simulink model "untitled"  (R2016b)
settings: Solver=VariableStepAuto  StartTime=0.0  StopTime=10.0  RelTol=1e-3
settings Model: Creator=drazz  LastModifiedBy=drazz

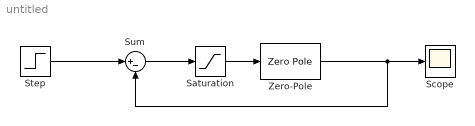
== system untitled ==
  Saturation : Saturate
  Scope : Scope
  Step : Step  SampleTime=0
  Sum : Sum  Inputs=|+-
  Zero-Pole : ZeroPole  Poles=[0 -1]
  wires:
  Zero-Pole/1 -> Sum/2, Scope/1
  Saturation/1 -> Zero-Pole/1
  Sum/1 -> Saturation/1
  Step/1 -> Sum/1
